simulink model "PitchController"  (R2024b)
settings: Solver=VariableStepAuto  StartTime=0.0  StopTime=10.0  RelTol=1e-3
libraries: cstblocks x1
settings Model: Creator=cpetr  LastModifiedBy=cpetr

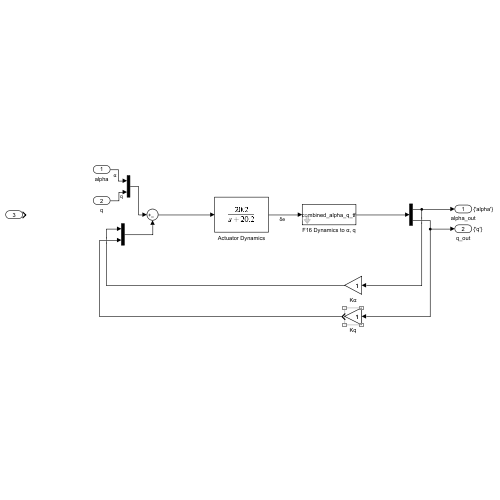
[thumbnail: Simulink's stored preview of the top-level diagram]
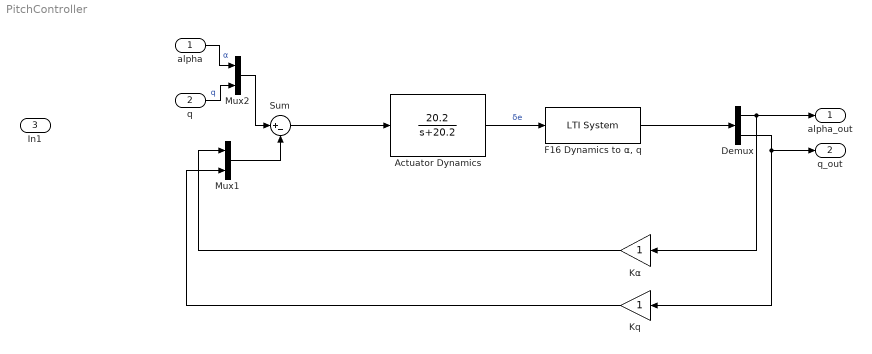
== system PitchController ==
  alpha : Inport
  q : Inport  Port=2
  In1 : Inport  Port=3
  Actuator Dynamics : TransferFcn  Numerator=[20.2]  Denominator=[1 20.2]  ContinuousStateAttributes={'alpha', 'q'}
  Demux : Demux  Outputs=2
  "F16 Dynamics to α, q" : cstblocks/LTI System  sys=combined_alpha_q_tf  IC=[]  PadeOrder=0
  Kq : Gain
  Kα : Gain
  Mux1 : Mux  Inputs=2
  Mux2 : Mux  Inputs=2
  Sum : Sum  Inputs=|+-
  alpha_out : Outport  SignalName={'alpha'}
  q_out : Outport  Port=2  SignalName={'q'}
  wires:
  Actuator Dynamics/1 -> "F16 Dynamics to α, q"/1  "δe"
  "F16 Dynamics to α, q"/1 -> Demux/1
  Demux/2 -> Kq/1, q_out/1
  Demux/1 -> Kα/1, alpha_out/1
  Kα/1 -> Mux1/1
  Mux1/1 -> Sum/2
  Mux2/1 -> Sum/1
  Sum/1 -> Actuator Dynamics/1
  Kq/1 -> Mux1/2
  alpha/1 -> Mux2/1  "α"
  q/1 -> Mux2/2  "q"
